simulink model "myfilenewest"  (R2022b)
settings: Solver=VariableStepAuto  StartTime=0.0  StopTime=90  RelTol=1e-3
settings Model: Creator=liqui  LastModifiedBy=liqui
settings OptimizationCC: UseDivisionForNetSlopeComputation=on

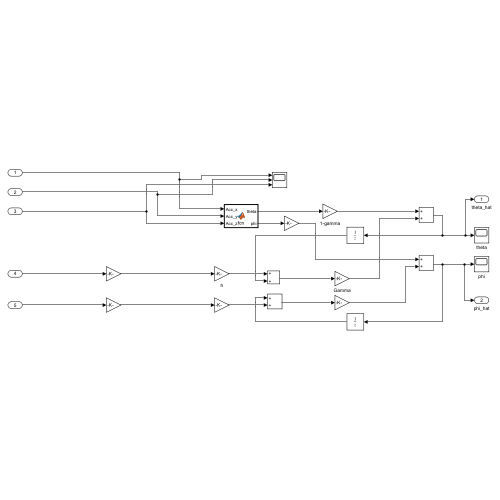
[thumbnail: Simulink's stored preview of the top-level diagram]
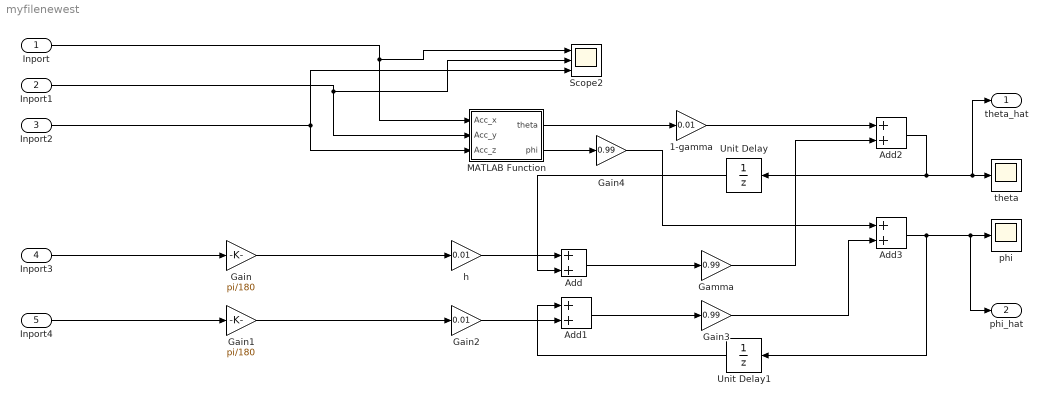
== system myfilenewest ==
  Inport : Inport
  Inport1 : Inport  Port=2
  Inport2 : Inport  Port=3
  Inport3 : Inport  Port=4
  Inport4 : Inport  Port=5
  1-gamma : Gain  Gain=0.01
  Add{,1..3} (4 alike) : Sum
  Gain : Gain  Gain=pi/180
  Gain1 : Gain  Gain=pi/180
  Gain2 : Gain  Gain=0.01
  Gain3 : Gain  Gain=0.99
  Gain4 : Gain  Gain=0.99
  Gamma : Gain  Gain=0.99
  MATLAB Function : MATLAB Function  TreatAsAtomicUnit=on
  Scope2 : Scope  NumInputPorts=3
  Unit Delay : UnitDelay  SampleTime=-1  HasFrameUpgradeWarning=on
  Unit Delay1 : UnitDelay  SampleTime=-1  HasFrameUpgradeWarning=on
  h : Gain  Gain=0.01
  phi : Scope
  theta : Scope
  theta_hat : Outport
  phi_hat : Outport  Port=2
  wires:
  MATLAB Function/1(theta) -> 1-gamma/1
  Gain/1 -> h/1
  Inport3/1 -> Gain/1
  Inport/1 -> Scope2/1, MATLAB Function/1(Acc_x)
  1-gamma/1 -> Add2/1
  Gamma/1 -> Add2/2
  Add2/1 -> theta_hat/1, theta/1, Unit Delay/1
  Add/1 -> Gamma/1
  Inport2/1 -> MATLAB Function/3(Acc_z), Scope2/3
  h/1 -> Add/1
  Inport1/1 -> MATLAB Function/2(Acc_y), Scope2/2
  MATLAB Function/2(phi) -> Gain4/1
  Inport4/1 -> Gain1/1
  Gain1/1 -> Gain2/1
  Gain2/1 -> Add1/2
  Add1/1 -> Gain3/1
  Gain4/1 -> Add3/1
  Gain3/1 -> Add3/2
  Add3/1 -> Unit Delay1/1, phi_hat/1, phi/1
  Unit Delay/1 -> Add/2
  Unit Delay1/1 -> Add1/1

== matlab function myfilenewest/MATLAB Function ==
  data: Acc_x input; theta output; Acc_y input; Acc_z input; phi output
function [theta,phi] = fcn(Acc_x,Acc_y,Acc_z)

theta=atan2(-Acc_x,sqrt(Acc_y.^2+Acc_z.^2));
phi = atan2(Acc_y,Acc_z);

end
